simulink model "entire_model"  (R2023b)
settings: Solver=VariableStepAuto  StartTime=0.0  StopTime=45  RelTol=1e-3
values from neighbouring files (symbols this model uses):
  b = [0 ... (first row only)    [CA3_params.m]
  b_bar = [1; 0]    [CA3_params_integral.m]
  g = K/tau    (= 24.8)    [CA3_params.m]    (also in CA3_params_integral.m; CA3_params_yp.m)
  Gamma = [100 0; 0  2000]    [CA3_params.m]    (also in CA3_params_integral.m = [gamma_y 0; 0  gamma_I])
  gamma = 125    [CA3_params.m]
  gamma_I = 1.0    (= 1)    [CA3_params_integral.m]
  gamma_r = 25    [CA3_params_yp.m]
  gamma_y = 1.0    (= 1)    [CA3_params_integral.m]    (also in CA3_params_yp.m = 25)
  P = lyap(Am', Q)    [CA3_params.m]
  P_bar = lyap(Am_bar, Q)    [CA3_params_integral.m]
libraries: matrix_library x7
settings Model: Creator=john  LastModifiedBy=john

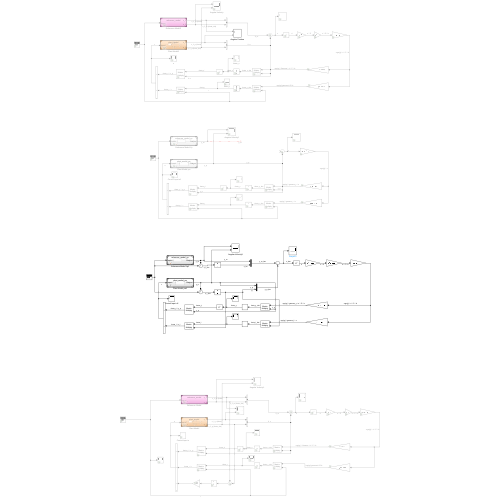
[thumbnail: Simulink's stored preview of the top-level diagram]
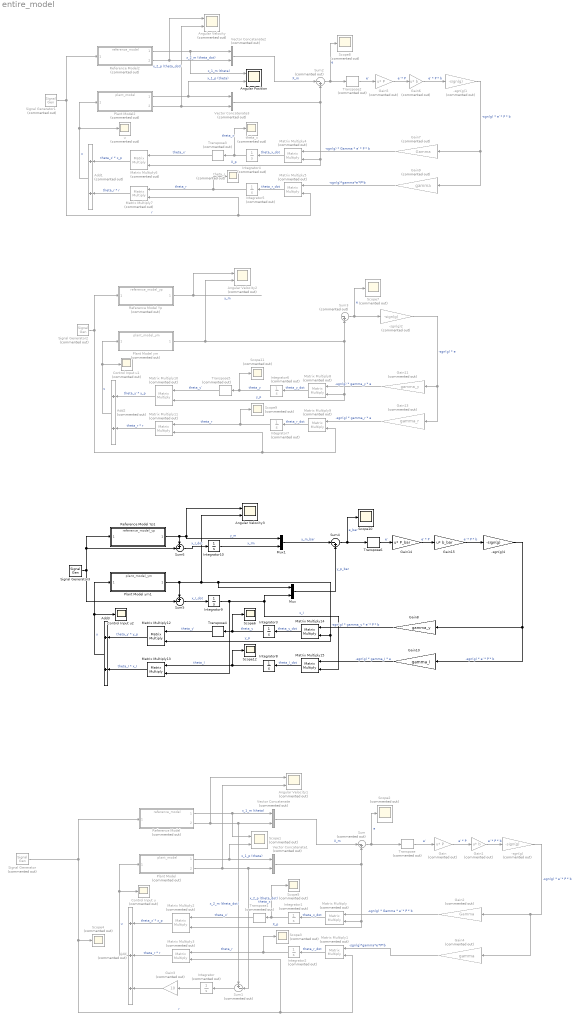
== system entire_model ==
  -sgn(g) : Gain  Commented=on  Gain=-sign(g)
  -sgn(g)1 : Gain  Commented=on  Gain=-sign(g)
  -sgn(g)2 : Gain  Commented=on  Gain=-sign(g)
  -sgn(g)4 : Gain  Gain=-sign(g)
  Add : Sum  Commented=on  Inputs=+++
  Add1 : Sum  Commented=on
  Add2 : Sum  Commented=on
  Add3 : Sum
  Angular Position : Scope  NumInputPorts=2
  Angular Velocity : Scope  Commented=on  NumInputPorts=2
  Angular Velocity1 : Scope  Commented=on  NumInputPorts=2
  Angular Velocity2 : Scope  Commented=on  NumInputPorts=2
  Angular Velocity3 : Scope  NumInputPorts=2
  Control Input u : Scope  Commented=on
  Control Input u1 : Scope  Commented=on
  Control Input u2 : Scope
  Gain : Gain  Commented=on  Gain=P  Multiplication=Matrix(u*K)
  Gain1 : Gain  Commented=on  Gain=b  Multiplication=Matrix(u*K)
  Gain10 : Gain  Gain=gamma_I
  Gain11 : Gain  Commented=on  Gain=gamma_y
  Gain13 : Gain  Commented=on  Gain=gamma_r
  Gain14 : Gain  Gain=P_bar  Multiplication=Matrix(u*K)
  Gain15 : Gain  Gain=b_bar  Multiplication=Matrix(u*K)
  Gain2 : Gain  Commented=on  Gain=Gamma
  Gain3 : Gain  Commented=on  Gain=10
  Gain4 : Gain  Commented=on  Gain=gamma
  Gain5 : Gain  Commented=on  Gain=P  Multiplication=Matrix(u*K)
  Gain6 : Gain  Commented=on  Gain=b  Multiplication=Matrix(u*K)
  Gain7 : Gain  Commented=on  Gain=Gamma
  Gain8 : Gain  Gain=gamma_y
  Gain9 : Gain  Commented=on  Gain=gamma
  Integrator{,1..2,4..7} (7 alike) : Integrator  Commented=on
  Integrator{3,8..10} (4 alike) : Integrator
  Matrix Multiply{,1..11} (12 alike) : Product  Commented=on  Multiplication=Matrix(*)
  Matrix Multiply{12..15} (4 alike) : Product  Multiplication=Matrix(*)
  Mux : Mux  Inputs=2
  Mux1 : Mux  Inputs=2
  Plant Model : ModelReference  Commented=on  ModelNameDialog=plant_model.slx  SimulationMode=Normal  ModelReferenceVersion=1.20
  Plant Model ym : ModelReference  Commented=on  ModelNameDialog=plant_model_ym.slx  SimulationMode=Normal  ModelReferenceVersion=1.2
  Plant Model ym1 : ModelReference  ModelNameDialog=plant_model_ym.slx  SimulationMode=Normal  ModelReferenceVersion=1.2
  Plant Model2 : ModelReference  Commented=on  ModelNameDialog=plant_model.slx  SimulationMode=Normal  ModelReferenceVersion=1.20
  Reference Model : ModelReference  Commented=on  ModelNameDialog=reference_model.slx  SimulationMode=Normal  ModelReferenceVersion=1.10
  Reference Model Yp : ModelReference  Commented=on  ModelNameDialog=reference_model_yp.slx  SimulationMode=Normal  ModelReferenceVersion=1.3
  Reference Model Yp1 : ModelReference  ModelNameDialog=reference_model_yp.slx  SimulationMode=Normal  ModelReferenceVersion=1.3
  Reference Model2 : ModelReference  Commented=on  ModelNameDialog=reference_model.slx  SimulationMode=Normal  ModelReferenceVersion=1.10
  Scope1 : Scope  Commented=on  NumInputPorts=2
  Scope10 : Scope
  Scope{2..5,7..9,11} (8 alike) : Scope  Commented=on
  Scope12 : Scope
  Scope6 : Scope
  Signal Generator : SignalGenerator  Commented=on  WaveForm=square  Units=rad/sec
  Signal Generator1 : SignalGenerator  Commented=on  WaveForm=square  Units=rad/sec
  Signal Generator2 : SignalGenerator  Commented=on  WaveForm=sawtooth  Units=rad/sec
  Signal Generator3 : SignalGenerator  WaveForm=sawtooth  Units=rad/sec
  Sum : Sum  Commented=on  Inputs=|-+
  Sum1 : Sum  Commented=on  Inputs=+-|
  Sum2 : Sum  Commented=on  Inputs=|-+
  Sum3 : Sum  Commented=on  Inputs=|-+
  Sum4 : Sum  Inputs=|-+
  Sum5 : Sum  Inputs=+-|
  Sum6 : Sum  Inputs=+-|
  Transpose{,1..3,5} (5 alike) : matrix_library/Transpose  Commented=on
  Transpose4 : matrix_library/Transpose
  Transpose6 : matrix_library/Transpose
  Vector Concatenate{,1..3} (4 alike) : Concatenate  Commented=on
  theta_r : Scope  Commented=on
  theta_x : Scope  Commented=on
  u : Scope  Commented=on
  wires:
  Reference Model/1 -> Scope1/1, Vector Concatenate/1  "x_1_m (theta)"
  Reference Model/2 -> Angular Velocity1/1, Sum1/1, Vector Concatenate/2  "x_2_m (theta_dot)"
  Plant Model/1 -> Vector Concatenate1/1, Scope1/2  "x_1_p (theta)"
  Plant Model/2 -> Angular Velocity1/2, Sum1/2, Vector Concatenate1/2  "x_2_p (theta_dot)"
  Gain/1 -> Gain1/1  "e' * P"
  Gain1/1 -> -sgn(g)/1  "e' * P * b"
  -sgn(g)/1 -> Gain4/1, Gain2/1  "-sgn(g) * e' * P * b"
  Vector Concatenate/1 -> Sum/1  "X_m"
  Sum/1 -> Transpose/1, Scope2/1  "e"
  Vector Concatenate1/1 -> Matrix Multiply/2, Matrix Multiply2/2, Sum/2  "X_p"
  Gain4/1 -> Matrix Multiply1/1  "-sgn(g)*gamma*e'*P*b"
  Matrix Multiply2/1 -> Add/1  "theta_x' * x_p"
  Matrix Multiply3/1 -> Add/2  "theta_r * r"
  Matrix Multiply1/1 -> Integrator2/1  "theta_r_dot"
  Integrator2/1 -> Scope3/1, Matrix Multiply3/1  "theta_r"
  Add/1 -> Control Input u/1, Plant Model/1  "u"
  Integrator1/1 -> Scope5/1, Transpose1/1  "theta_x"
  Transpose1/1 -> Matrix Multiply2/1  "theta_x'"
  Transpose/1 -> Gain/1  "e'"
  Matrix Multiply/1 -> Integrator1/1  "theta_x_dot"
  Gain2/1 -> Matrix Multiply/1  "-sgn(g) * Gamma * e' * P * b"
  Integrator/1 -> Gain3/1
  Signal Generator/1 -> Reference Model/1, Scope4/1, Matrix Multiply3/2, Matrix Multiply1/2  "r"
  Sum1/1 -> Integrator/1
  Gain3/1 -> Add/3
  Integrator5/1 -> theta_r/1, Matrix Multiply7/1  "theta_r"
  Integrator4/1 -> theta_x/1, Transpose3/1  "theta_x"
  Vector Concatenate3/1 -> Matrix Multiply4/2, Matrix Multiply6/2, Sum2/2  "X_p"
  Matrix Multiply6/1 -> Add1/1  "theta_x' * x_p"
  Matrix Multiply7/1 -> Add1/2  "theta_r * r"
  Matrix Multiply5/1 -> Integrator5/1  "theta_r_dot"
  Plant Model2/1 -> Vector Concatenate3/1, Angular Position/2  "x_1_p (theta)"
  Sum2/1 -> Transpose2/1, Scope8/1  "e"
  Gain5/1 -> Gain6/1  "e' * P"
  Transpose2/1 -> Gain5/1  "e'"
  Transpose3/1 -> Matrix Multiply6/1  "theta_x'"
  Gain7/1 -> Matrix Multiply4/1  "-sgn(g) * Gamma * e' * P * b"
  Gain6/1 -> -sgn(g)1/1  "e' * P * b"
  Vector Concatenate2/1 -> Sum2/1  "X_m"
  Plant Model2/2 -> Angular Velocity/2, Vector Concatenate3/2  "x_2_p (theta_dot)"
  Reference Model2/2 -> Vector Concatenate2/2, Angular Velocity/1  "x_2_m (theta_dot)"
  Matrix Multiply4/1 -> Integrator4/1  "theta_x_dot"
  Reference Model2/1 -> Angular Position/1, Vector Concatenate2/1  "x_1_m (theta)"
  Add1/1 -> u/1, Plant Model2/1  "u"
  Signal Generator1/1 -> Reference Model2/1, Matrix Multiply5/2, Matrix Multiply7/2  "r"
  Gain9/1 -> Matrix Multiply5/1  "-sgn(g)*gamma*e'*P*b"
  -sgn(g)1/1 -> Gain9/1, Gain7/1  "-sgn(g) * e' * P * b"
  Matrix Multiply10/1 -> Add2/1  "theta_y' * y_p"
  Matrix Multiply9/1 -> Integrator7/1  "theta_r_dot"
  Sum3/1 -> -sgn(g)2/1, Scope7/1  "e"
  Integrator7/1 -> Scope9/1, Matrix Multiply11/1  "theta_r"
  Reference Model Yp/1 -> Angular Velocity2/1  "y_m"
  -sgn(g)2/1 -> Gain13/1, Gain11/1  "-sgn(g) * e"
  Signal Generator2/1 -> Reference Model Yp/1, Matrix Multiply9/2, Matrix Multiply11/2
  Add2/1 -> Plant Model ym/1, Control Input u1/1  "u"
  Transpose5/1 -> Matrix Multiply10/1  "theta_y'"
  Gain11/1 -> Matrix Multiply8/1  "-sgn(g) * gamma_y * e"
  Integrator6/1 -> Scope11/1, Transpose5/1  "theta_y"
  Gain13/1 -> Matrix Multiply9/1  "-sgn(g) * gamma_r * e"
  Matrix Multiply8/1 -> Integrator6/1  "theta_y_dot"
  Plant Model ym/1 -> Angular Velocity2/2, Sum3/2, Matrix Multiply8/2, Matrix Multiply10/2  "y_p"
  Matrix Multiply11/1 -> Add2/2  "theta_r * r"
  Matrix Multiply15/1 -> Integrator8/1  "theta_I_dot"
  Sum4/1 -> Transpose6/1, Scope10/1  "e_bar"
  Gain10/1 -> Matrix Multiply15/1  "-sgn(g) * gamma_I * e"
  Matrix Multiply13/1 -> Add3/2  "theta_I * x_I"
  Gain8/1 -> Matrix Multiply14/1  "-sgn(g) * gamma_y * e' * P * b"
  Add3/1 -> Plant Model ym1/1, Control Input u2/1  "u"
  Reference Model Yp1/1 -> Sum6/1, Mux1/1, Angular Velocity3/1  "y_m"
  Integrator8/1 -> Scope12/1, Matrix Multiply13/1  "theta_I"
  Plant Model ym1/1 -> Mux/1, Matrix Multiply12/2, Matrix Multiply14/2, Angular Velocity3/2, Sum5/1  "y_p"
  Transpose4/1 -> Matrix Multiply12/1  "theta_y'"
  Signal Generator3/1 -> Sum5/2, Reference Model Yp1/1, Sum6/2
  Matrix Multiply12/1 -> Add3/1  "theta_y' * y_p"
  Matrix Multiply14/1 -> Integrator3/1  "theta_y_dot"
  Integrator3/1 -> Scope6/1, Transpose4/1  "theta_y"
  Sum5/1 -> Integrator9/1  "x_I_dot"
  Integrator9/1 -> Matrix Multiply13/2, Mux/2, Matrix Multiply15/2  "x_I"
  -sgn(g)4/1 -> Gain8/1, Gain10/1  "-sgn(g) * e' * P * b"
  Gain15/1 -> -sgn(g)4/1  "e' * P * b"
  Transpose6/1 -> Gain14/1  "e'"
  Gain14/1 -> Gain15/1  "e' * P"
  Integrator10/1 -> Mux1/2  "x_Im"
  Sum6/1 -> Integrator10/1  "x_I_dot"
  Mux/1 -> Sum4/2  "y_p_bar"
  Mux1/1 -> Sum4/1  "y_m_bar"
